simulink library "albedo_lib"  (Simulink 6.2)
undefined symbols (not defined in the file or in its folder): albedo_path, albedo_wrapper, filesep, Ts
settings Model: LastModifiedBy=Martin

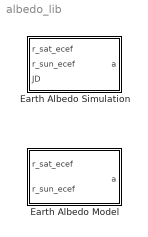
== system albedo_lib ==
  Earth Albedo Model : Subsystem  TreatAsAtomicUnit=on  mask(Earth Albedo Model){eprdata=load('lib/space_environment_emulation/albedo/toolbox/epr_data/2003/ga030101-031231'), redfac=1, Ts=1, enable=on}
      mask prompts: eprdata "Reflectivity Data (EPR Struct):"; redfac "Reduction factor:"; Ts "Sample Time (-1 for inherited):"
      mask help: Calculate Earth Albedo using static data from the EP/TOMS spacecraft.
      mask init:
      | global sy;
      | global sx;
      | sy = round(180/redfac);
      | sx = round(288/redfac);
      mask Help:
      | <b>Input</b><br>
      | Sat: Vector to satellite in ECEF [m]<br>
      | Sun: Vector to the Sun in ECEF [m]<p>
      | <b>Parameters</b><br>
      | Reflectivity Data (EPR Struct): TOMS Reflectivity data [E.U].<br>
      | Reduction factor: Reduce data resolution by this factor.<br>
      | Sample Time (-1 for inherited): Sample Time [s]. The block cannot inherit continuous sample time.<br>
      | Enable: Enable or disable albedo calculation<p>
      | <b>Output</b><br>
      | Albedo: Fraction of solar irradiance received on the satellite. The incoming solar irradiance is 1366.5 W/m^2<p>
      mask CallbackString: |||enable = strcmp(get_param(gcb,'enable'),'on');
      mask Display:
      | image(imread('private/albedoicon.png'));
      | port_label('output', 1, 'Albedo');
      | port_label('input', 1, 'Sat');
      | port_label('input', 2, 'Sun');
  Earth Albedo Simulation : Subsystem  TreatAsAtomicUnit=on  mask(Earth Albedo Simuation){pathstr=[albedo_path filesep 'epr_data'], redfac=4, Ts=Ts, enable=off}
      mask prompts: pathstr "Path to reflectivity data directories:"; redfac "Reduction factor:"; Ts "Sample Time (-1 for inherited):"
      mask help: Calculate Earth Albedo using daily reflectivity data from the EP/TOMS spacecraft.
      mask init:
      | global sy;
      | global sx;
      | sy = round(180/redfac);
      | sx = round(288/redfac);
      mask Help:
      | <b>Input</b><br>
      | Sat: Vector to satellite in ECEF [m]<br>
      | Sun: Vector to the Sun in ECEF [m]<br>
      | Time: Time in Julian Date [days]<p>
      | <b>Parameters</b><br>
      | Path to reflectivity data directories: System path to TOMS Earth Reflectivity Data. The data must be structured in i directiry for each year. The path is searched for the newest data, determined from the Time input.<br>
      | Reduction factor: Reduce data resolution by this factor.<br>
      | Sample Time (-1 for inherited): Sample Time [s]. The block cannot inherit continuous sample time.<br>
      | Enable: Enable or disable albedo calculation<p>
      | <b>Output</b><br>
      | Albedo: Fraction of solar irradiance received on the satellite. The incoming solar irradiance is 1366.5 W/m^2<p>
      mask CallbackString: |||enable = strcmp(get_param(gcb,'enable'),'on');
      mask Display:
      | image(imread('private/albedoicon.png'));
      | port_label('output', 1, 'Albedo');
      | port_label('input', 1, 'Sat');
      | port_label('input', 2, 'Sun');
      | port_label('input', 3, 'Time');

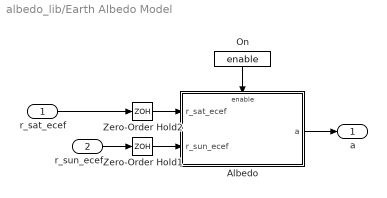
== system albedo_lib/Earth Albedo Model ==
  r_sat_ecef : Inport  Port=1  SampleTime=Ts  LatchInput=off
  r_sun_ecef : Inport  Port=2  SampleTime=Ts  LatchInput=off
  Albedo : Subsystem
  On : Constant  Orientation=down  Value=enable
  Zero-Order Hold1 : ZeroOrderHold  SampleTime=Ts
  Zero-Order Hold2 : ZeroOrderHold  SampleTime=Ts
  a : Outport
  wires:
  On/1 -> Albedo/Enable
  r_sat_ecef/1 -> Zero-Order Hold2/1
  Albedo/1(a) -> a/1
  r_sun_ecef/1 -> Zero-Order Hold1/1
  Zero-Order Hold2/1 -> Albedo/1(r_sat_ecef)
  Zero-Order Hold1/1 -> Albedo/2(r_sun_ecef)

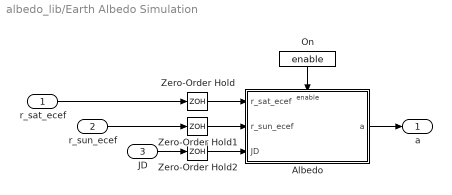
== system albedo_lib/Earth Albedo Simulation ==
  r_sat_ecef : Inport  Port=1  PortDimensions=3  SampleTime=Ts  LatchInput=off
  r_sun_ecef : Inport  Port=2  PortDimensions=3  SampleTime=Ts  LatchInput=off
  JD : Inport  Port=3  PortDimensions=1  SampleTime=Ts  LatchInput=off
  Albedo : Subsystem
  On : Constant  Orientation=down  Value=enable
  Zero-Order Hold : ZeroOrderHold  SampleTime=Ts
  Zero-Order Hold1 : ZeroOrderHold  SampleTime=Ts
  Zero-Order Hold2 : ZeroOrderHold  SampleTime=Ts
  a : Outport
  wires:
  r_sun_ecef/1 -> Zero-Order Hold1/1
  Albedo/1(a) -> a/1
  r_sat_ecef/1 -> Zero-Order Hold/1
  On/1 -> Albedo/Enable
  JD/1 -> Zero-Order Hold2/1
  Zero-Order Hold/1 -> Albedo/1(r_sat_ecef)
  Zero-Order Hold1/1 -> Albedo/2(r_sun_ecef)
  Zero-Order Hold2/1 -> Albedo/3(JD)

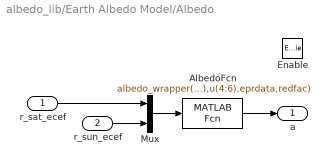
== system albedo_lib/Earth Albedo Model/Albedo ==
  r_sat_ecef : Inport  Port=1  PortDimensions=3  LatchInput=off
  r_sun_ecef : Inport  Port=2  PortDimensions=3  LatchInput=off
  Enable : EnablePort  StatesWhenEnabling=reset
  AlbedoFcn : MATLABFcn  MATLABFcn=albedo_wrapper(u(1:3),u(4:6),eprdata,redfac)  OutputDimensions=floor([180 288]./redfac)  OutputSignalType=real  Output1D=off
  Mux : Mux  Inputs=2
  a : Outport  OutputWhenDisabled=reset  InitialOutput=0
  wires:
  r_sun_ecef/1 -> Mux/2
  AlbedoFcn/1 -> a/1
  r_sat_ecef/1 -> Mux/1
  Mux/1 -> AlbedoFcn/1

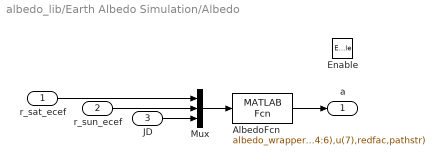
== system albedo_lib/Earth Albedo Simulation/Albedo ==
  r_sat_ecef : Inport  Port=1  PortDimensions=3  LatchInput=off
  r_sun_ecef : Inport  Port=2  PortDimensions=3  LatchInput=off
  JD : Inport  Port=3  PortDimensions=1  LatchInput=off
  Enable : EnablePort  StatesWhenEnabling=reset
  AlbedoFcn : MATLABFcn  MATLABFcn=albedo_wrapper(u(1:3),u(4:6),u(7),redfac,pathstr)  OutputDimensions=floor([180 288]./redfac)  OutputSignalType=real  Output1D=off
  Mux : Mux  Inputs=3
  a : Outport  OutputWhenDisabled=reset  InitialOutput=0
  wires:
  Mux/1 -> AlbedoFcn/1
  r_sat_ecef/1 -> Mux/1
  AlbedoFcn/1 -> a/1
  r_sun_ecef/1 -> Mux/2
  JD/1 -> Mux/3
